simulink model "final simulation file"  (R2021a)
settings: Solver=ode8  StartTime=0.0  StopTime=0.1  FixedStep=1e-7  RelTol=1e-3
undefined symbols (not defined in the file): Acid, Lead
libraries: spsSeriesRLCBranchLib x13, spsIGBTLib x6, pid_lib x4, sldrtlib x4, spsAlphaBetaZerotodq0Lib x2, simulink x2, spsThreePhaseVIMeasurementLib x2, spsDiodeLib x1, spsIdealSwitchLib x1, spsMosfetLib x1, spsPower3phInstantaneousLib x1, spsBatteryLib x1
settings Model: Creator=RISHABH KUMAR  LastModifiedBy=RISHABH KUMAR

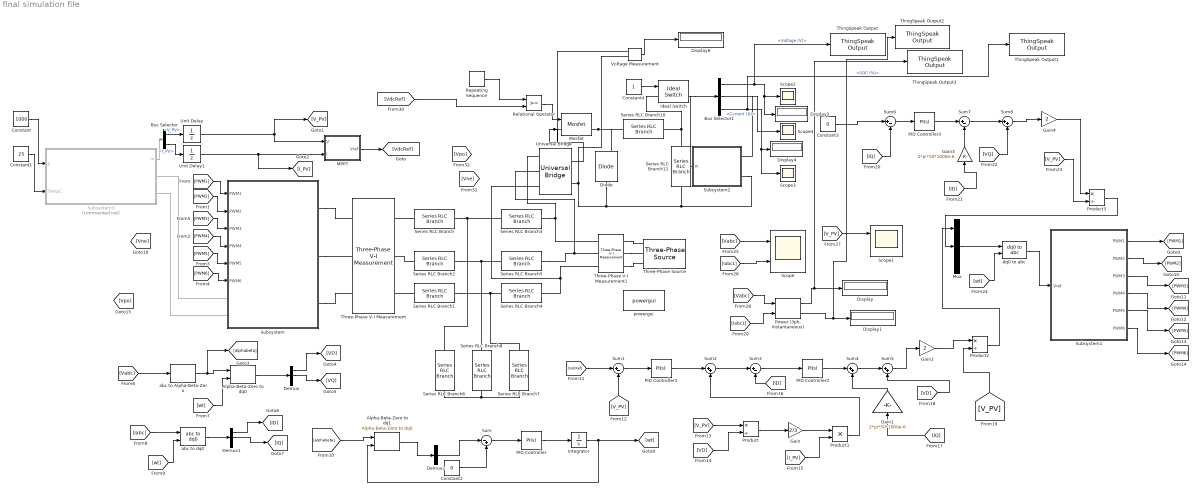
== system final simulation file ==
  Alpha-Beta-Zero to dq0 : spsAlphaBetaZerotodq0Lib/Alpha-Beta-Zero to dq0  Alignment=90 degrees behind phase A axis
      settings: SourceProductBaseCode=PS
  Alpha-Beta-Zero to dq1 : spsAlphaBetaZerotodq0Lib/Alpha-Beta-Zero to dq0  Alignment=90 degrees behind phase A axis
      settings: SourceProductBaseCode=PS
  Bus Selector : BusSelector  OutputSignals=V_PV,I_PV
  Bus Selector1 : BusSelector  OutputSignals=Voltage (V),Current (A),SOC (%)
  Constant : Constant  Value=1000
  Constant1 : Constant  Value=25
  Constant2 : Constant  Value=0
  Constant3 : Constant  Value=0
  Constant4 : Constant
  Demux : Demux  Outputs=3
  Demux1 : Demux  Outputs=3
  Demux2 : Demux  Outputs=3
  Diode : spsDiodeLib/Diode  Ron=0.001  Lon=0  Vf=0.8  IC=0  UseSnubber=0  Rs=500  Cs=250e-9  Measurements=on
  Display{,1..2,4,6} (5 alike) : Display
  Gain : Gain  Gain=2/3
  Gain1 : Gain  Gain=2*pi*50*1000e-6
  Gain2 : Gain  Gain=2
  Gain3 : Gain  Gain=2*pi*50*1000e-6
  Gain4 : Gain  Gain=2
  Ideal Switch : spsIdealSwitchLib/Ideal Switch  Ron=0.00001  Lon=0  IC=0  Rs=1e5  Cs=inf  Measurements=on
  Integrator : Integrator
  MPPT : MATLAB Function  TreatAsAtomicUnit=on
  Mosfet : spsMosfetLib/Mosfet  Ron=0.1  Lon=0  Rd=0.01  Vfd=0  IC=0  Rs=1e5  Cs=inf  Measurements=on
  Mux : Mux  Inputs=3
  PID Controller : pid_lib/PID Controller  Controller=PI  Form=Parallel  TimeDomain=Continuous-time  UseExternalTs=off  SampleTime=-1  IntegratorMethod=Forward Euler  FilterMethod=Forward Euler  ControllerParametersSource=internal  P=10  I=50000  D=0  UseFilter=on  N=100  TunerSelectOption=Transfer Function Based (PID Tuner App)  InitialConditionSource=internal  InitialConditionForIntegrator=0  InitialConditionForFilter=0  DifferentiatorICPrevScaledInput=0  ExternalReset=none  TrackingMode=off  Kt=1  LimitOutput=off  SatLimitsSource=internal  UpperSaturationLimit=inf  LowerSaturationLimit=-inf  LinearizeAsGain=on  AntiWindupMode=none  Kb=1  POutMin=[]  POutMax=[]  IOutMin=[]  IOutMax=[]  DOutMin=[]  DOutMax=[]  NOutMin=[]  NOutMax=[]  SumOutMin=[]  SumOutMax=[]  SaturationOutMin=[]  SaturationOutMax=[]  PParamMin=[]  PParamMax=[]  IParamMin=[]  IParamMax=[]  DParamMin=[]  DParamMax=[]  NParamMin=[]  NParamMax=[]  KbParamMin=[]  KbParamMax=[]  KtParamMin=[]  KtParamMax=[]  KbOutMin=[]  KbOutMax=[]  KtOutMin=[]  KtOutMax=[]  IntegratorOutMin=[]  IntegratorOutMax=[]  FilterOutMin=[]  FilterOutMax=[]  SumI1OutMin=[]  SumI1OutMax=[]  SumI2OutMin=[]  SumI2OutMax=[]  SumI3OutMin=[]  SumI3OutMax=[]  SumI4OutMin=[]  SumI4OutMax=[]  SumDOutMin=[]  SumDOutMax=[]  DifferentiatorOutMin=[]  DifferentiatorOutMax=[]  FilterDiffOutCoefMin=[]  FilterDiffOutCoefMax=[]  ReciprocalOutMin=[]  ReciprocalOutMax=[]  SumDenOutMin=[]  SumDenOutMax=[]  SumNumOutMin=[]  SumNumOutMax=[]  DivideOutMin=[]  DivideOutMax=[]  UdiffTsProdOutMin=[]  UdiffTsProdOutMax=[]  NTsProdOutMin=[]  NTsProdOutMax=[]  UintegralTsProdOutMin=[]  UintegralTsProdOutMax=[]  UngainTsProdOutMin=[]  UngainTsProdOutMax=[]  IntegratorContinuousStateAttributes=''  IntegratorStateMustResolveToSignalObject=off  IntegratorRTWStateStorageClass=Auto  FilterContinuousStateAttributes=''  FilterStateMustResolveToSignalObject=off  FilterRTWStateStorageClass=Auto  ParallelPVariant=InternalParameters  IdealPVariant=Disabled  IVariant=InternalParameters  DVariant=Disabled  IntegratorVariant=Continuous  SatVariant=Disabled  AWVariant=Passthrough  PCopyVariant=Disabled  TRVariant=Disabled  FdbkBlocksVariant=Forward  IdealPFdbkVariant=Disabled  SatFdbkVariant=Disabled  DerivativeFilterVariant=Disabled  NVariant=Disabled  NCopyVariant=Disabled_SignalSpec  FilterICVariant=Disabled  IntegratorICVariant=InternalICs  ExternalResetVariant=Disabled  TRSumVariant=Passthrough  SumFdbkVariant=Disabled  SumVariant=Sum_PI  TsampFilterVariant=InternalTs  TsampNgainVariant=Passthrough  TsampIntegralVariant=Passthrough  ExternalSaturationOutDataTypeStr=Inherit: Same as second input
  PID Controller1 : pid_lib/PID Controller  Controller=PI  Form=Parallel  TimeDomain=Continuous-time  UseExternalTs=off  SampleTime=-1  IntegratorMethod=Forward Euler  FilterMethod=Forward Euler  ControllerParametersSource=internal  P=0.25  I=0.001  D=0  UseFilter=on  N=100  TunerSelectOption=Transfer Function Based (PID Tuner App)  InitialConditionSource=internal  InitialConditionForIntegrator=0  InitialConditionForFilter=0  DifferentiatorICPrevScaledInput=0  ExternalReset=none  TrackingMode=off  Kt=1  LimitOutput=off  SatLimitsSource=internal  UpperSaturationLimit=inf  LowerSaturationLimit=-inf  LinearizeAsGain=on  AntiWindupMode=none  Kb=1  POutMin=[]  POutMax=[]  IOutMin=[]  IOutMax=[]  DOutMin=[]  DOutMax=[]  NOutMin=[]  NOutMax=[]  SumOutMin=[]  SumOutMax=[]  SaturationOutMin=[]  SaturationOutMax=[]  PParamMin=[]  PParamMax=[]  IParamMin=[]  IParamMax=[]  DParamMin=[]  DParamMax=[]  NParamMin=[]  NParamMax=[]  KbParamMin=[]  KbParamMax=[]  KtParamMin=[]  KtParamMax=[]  KbOutMin=[]  KbOutMax=[]  KtOutMin=[]  KtOutMax=[]  IntegratorOutMin=[]  IntegratorOutMax=[]  FilterOutMin=[]  FilterOutMax=[]  SumI1OutMin=[]  SumI1OutMax=[]  SumI2OutMin=[]  SumI2OutMax=[]  SumI3OutMin=[]  SumI3OutMax=[]  SumI4OutMin=[]  SumI4OutMax=[]  SumDOutMin=[]  SumDOutMax=[]  DifferentiatorOutMin=[]  DifferentiatorOutMax=[]  FilterDiffOutCoefMin=[]  FilterDiffOutCoefMax=[]  ReciprocalOutMin=[]  ReciprocalOutMax=[]  SumDenOutMin=[]  SumDenOutMax=[]  SumNumOutMin=[]  SumNumOutMax=[]  DivideOutMin=[]  DivideOutMax=[]  UdiffTsProdOutMin=[]  UdiffTsProdOutMax=[]  NTsProdOutMin=[]  NTsProdOutMax=[]  UintegralTsProdOutMin=[]  UintegralTsProdOutMax=[]  UngainTsProdOutMin=[]  UngainTsProdOutMax=[]  IntegratorContinuousStateAttributes=''  IntegratorStateMustResolveToSignalObject=off  IntegratorRTWStateStorageClass=Auto  FilterContinuousStateAttributes=''  FilterStateMustResolveToSignalObject=off  FilterRTWStateStorageClass=Auto  ParallelPVariant=InternalParameters  IdealPVariant=Disabled  IVariant=InternalParameters  DVariant=Disabled  IntegratorVariant=Continuous  SatVariant=Disabled  AWVariant=Passthrough  PCopyVariant=Disabled  TRVariant=Disabled  FdbkBlocksVariant=Forward  IdealPFdbkVariant=Disabled  SatFdbkVariant=Disabled  DerivativeFilterVariant=Disabled  NVariant=Disabled  NCopyVariant=Disabled_SignalSpec  FilterICVariant=Disabled  IntegratorICVariant=InternalICs  ExternalResetVariant=Disabled  TRSumVariant=Passthrough  SumFdbkVariant=Disabled  SumVariant=Sum_PI  TsampFilterVariant=InternalTs  TsampNgainVariant=Passthrough  TsampIntegralVariant=Passthrough  ExternalSaturationOutDataTypeStr=Inherit: Same as second input
  PID Controller2 : pid_lib/PID Controller  Controller=PI  Form=Parallel  TimeDomain=Continuous-time  UseExternalTs=off  SampleTime=-1  IntegratorMethod=Forward Euler  FilterMethod=Forward Euler  ControllerParametersSource=internal  P=3.33  I=5000  D=0  UseFilter=on  N=100  TunerSelectOption=Transfer Function Based (PID Tuner App)  InitialConditionSource=internal  InitialConditionForIntegrator=0  InitialConditionForFilter=0  DifferentiatorICPrevScaledInput=0  ExternalReset=none  TrackingMode=off  Kt=1  LimitOutput=off  SatLimitsSource=internal  UpperSaturationLimit=inf  LowerSaturationLimit=-inf  LinearizeAsGain=on  AntiWindupMode=none  Kb=1  POutMin=[]  POutMax=[]  IOutMin=[]  IOutMax=[]  DOutMin=[]  DOutMax=[]  NOutMin=[]  NOutMax=[]  SumOutMin=[]  SumOutMax=[]  SaturationOutMin=[]  SaturationOutMax=[]  PParamMin=[]  PParamMax=[]  IParamMin=[]  IParamMax=[]  DParamMin=[]  DParamMax=[]  NParamMin=[]  NParamMax=[]  KbParamMin=[]  KbParamMax=[]  KtParamMin=[]  KtParamMax=[]  KbOutMin=[]  KbOutMax=[]  KtOutMin=[]  KtOutMax=[]  IntegratorOutMin=[]  IntegratorOutMax=[]  FilterOutMin=[]  FilterOutMax=[]  SumI1OutMin=[]  SumI1OutMax=[]  SumI2OutMin=[]  SumI2OutMax=[]  SumI3OutMin=[]  SumI3OutMax=[]  SumI4OutMin=[]  SumI4OutMax=[]  SumDOutMin=[]  SumDOutMax=[]  DifferentiatorOutMin=[]  DifferentiatorOutMax=[]  FilterDiffOutCoefMin=[]  FilterDiffOutCoefMax=[]  ReciprocalOutMin=[]  ReciprocalOutMax=[]  SumDenOutMin=[]  SumDenOutMax=[]  SumNumOutMin=[]  SumNumOutMax=[]  DivideOutMin=[]  DivideOutMax=[]  UdiffTsProdOutMin=[]  UdiffTsProdOutMax=[]  NTsProdOutMin=[]  NTsProdOutMax=[]  UintegralTsProdOutMin=[]  UintegralTsProdOutMax=[]  UngainTsProdOutMin=[]  UngainTsProdOutMax=[]  IntegratorContinuousStateAttributes=''  IntegratorStateMustResolveToSignalObject=off  IntegratorRTWStateStorageClass=Auto  FilterContinuousStateAttributes=''  FilterStateMustResolveToSignalObject=off  FilterRTWStateStorageClass=Auto  ParallelPVariant=InternalParameters  IdealPVariant=Disabled  IVariant=InternalParameters  DVariant=Disabled  IntegratorVariant=Continuous  SatVariant=Disabled  AWVariant=Passthrough  PCopyVariant=Disabled  TRVariant=Disabled  FdbkBlocksVariant=Forward  IdealPFdbkVariant=Disabled  SatFdbkVariant=Disabled  DerivativeFilterVariant=Disabled  NVariant=Disabled  NCopyVariant=Disabled_SignalSpec  FilterICVariant=Disabled  IntegratorICVariant=InternalICs  ExternalResetVariant=Disabled  TRSumVariant=Passthrough  SumFdbkVariant=Disabled  SumVariant=Sum_PI  TsampFilterVariant=InternalTs  TsampNgainVariant=Passthrough  TsampIntegralVariant=Passthrough  ExternalSaturationOutDataTypeStr=Inherit: Same as second input
  PID Controller3 : pid_lib/PID Controller  Controller=PI  Form=Parallel  TimeDomain=Continuous-time  UseExternalTs=off  SampleTime=-1  IntegratorMethod=Forward Euler  FilterMethod=Forward Euler  ControllerParametersSource=internal  P=3.33  I=5000  D=0  UseFilter=on  N=100  TunerSelectOption=Transfer Function Based (PID Tuner App)  InitialConditionSource=internal  InitialConditionForIntegrator=0  InitialConditionForFilter=0  DifferentiatorICPrevScaledInput=0  ExternalReset=none  TrackingMode=off  Kt=1  LimitOutput=off  SatLimitsSource=internal  UpperSaturationLimit=inf  LowerSaturationLimit=-inf  LinearizeAsGain=on  AntiWindupMode=none  Kb=1  POutMin=[]  POutMax=[]  IOutMin=[]  IOutMax=[]  DOutMin=[]  DOutMax=[]  NOutMin=[]  NOutMax=[]  SumOutMin=[]  SumOutMax=[]  SaturationOutMin=[]  SaturationOutMax=[]  PParamMin=[]  PParamMax=[]  IParamMin=[]  IParamMax=[]  DParamMin=[]  DParamMax=[]  NParamMin=[]  NParamMax=[]  KbParamMin=[]  KbParamMax=[]  KtParamMin=[]  KtParamMax=[]  KbOutMin=[]  KbOutMax=[]  KtOutMin=[]  KtOutMax=[]  IntegratorOutMin=[]  IntegratorOutMax=[]  FilterOutMin=[]  FilterOutMax=[]  SumI1OutMin=[]  SumI1OutMax=[]  SumI2OutMin=[]  SumI2OutMax=[]  SumI3OutMin=[]  SumI3OutMax=[]  SumI4OutMin=[]  SumI4OutMax=[]  SumDOutMin=[]  SumDOutMax=[]  DifferentiatorOutMin=[]  DifferentiatorOutMax=[]  FilterDiffOutCoefMin=[]  FilterDiffOutCoefMax=[]  ReciprocalOutMin=[]  ReciprocalOutMax=[]  SumDenOutMin=[]  SumDenOutMax=[]  SumNumOutMin=[]  SumNumOutMax=[]  DivideOutMin=[]  DivideOutMax=[]  UdiffTsProdOutMin=[]  UdiffTsProdOutMax=[]  NTsProdOutMin=[]  NTsProdOutMax=[]  UintegralTsProdOutMin=[]  UintegralTsProdOutMax=[]  UngainTsProdOutMin=[]  UngainTsProdOutMax=[]  IntegratorContinuousStateAttributes=''  IntegratorStateMustResolveToSignalObject=off  IntegratorRTWStateStorageClass=Auto  FilterContinuousStateAttributes=''  FilterStateMustResolveToSignalObject=off  FilterRTWStateStorageClass=Auto  ParallelPVariant=InternalParameters  IdealPVariant=Disabled  IVariant=InternalParameters  DVariant=Disabled  IntegratorVariant=Continuous  SatVariant=Disabled  AWVariant=Passthrough  PCopyVariant=Disabled  TRVariant=Disabled  FdbkBlocksVariant=Forward  IdealPFdbkVariant=Disabled  SatFdbkVariant=Disabled  DerivativeFilterVariant=Disabled  NVariant=Disabled  NCopyVariant=Disabled_SignalSpec  FilterICVariant=Disabled  IntegratorICVariant=InternalICs  ExternalResetVariant=Disabled  TRSumVariant=Passthrough  SumFdbkVariant=Disabled  SumVariant=Sum_PI  TsampFilterVariant=InternalTs  TsampNgainVariant=Passthrough  TsampIntegralVariant=Passthrough  ExternalSaturationOutDataTypeStr=Inherit: Same as second input
  "Power (3ph, Instantaneous)" : spsPower3phInstantaneousLib/Power (3ph, Instantaneous)
  Product : Product  Inputs=*/
  Product1 : Product
  Product2 : Product  Inputs=*/
  Product3 : Product  Inputs=*/
  Relational Operator : RelationalOperator  OutDataTypeStr=boolean  RndMeth=Simplest
  Repeating Sequence : simulink/Sources/Repeating Sequence  rep_seq_t=[0 0.0001]  rep_seq_y=[0 1]
  Scope : Scope  NumInputPorts=2
  Scope1 : Scope  NumInputPorts=2
  Scope2 : Scope
  Scope3 : Scope
  Scope4 : Scope
  Series RLC Branch{,1..5} (6 alike) : spsSeriesRLCBranchLib/Series RLC Branch  LConnTagsString=__new0  RConnTagsString=__new0  BranchType=RL  Resistance=1e-3  Inductance=500e-3  SetiL0=off  InitialCurrent=0  Capacitance=1e-6  Setx0=off  InitialVoltage=0  Measurements=None
  Series RLC Branch10 : spsSeriesRLCBranchLib/Series RLC Branch  LConnTagsString=__new0  RConnTagsString=__new0  BranchType=L  Resistance=1  Inductance=0.0417  SetiL0=off  InitialCurrent=0  Capacitance=1e-6  Setx0=off  InitialVoltage=0  Measurements=None
  Series RLC Branch11 : spsSeriesRLCBranchLib/Series RLC Branch  LConnTagsString=__new0  RConnTagsString=__new0  BranchType=C  Resistance=1  Inductance=0.783e-3  SetiL0=off  InitialCurrent=0  Capacitance=1.198e-3  Setx0=off  InitialVoltage=0  Measurements=None
  Series RLC Branch6 : spsSeriesRLCBranchLib/Series RLC Branch  LConnTagsString=__new0  RConnTagsString=__new0  BranchType=RC  Resistance=1e-3  Inductance=500e-3  SetiL0=off  InitialCurrent=0  Capacitance=100e-6  Setx0=off  InitialVoltage=0  Measurements=None
  Series RLC Branch7 : spsSeriesRLCBranchLib/Series RLC Branch  LConnTagsString=__new0  RConnTagsString=__new0  BranchType=RC  Resistance=1e-3  Inductance=500e-3  SetiL0=off  InitialCurrent=0  Capacitance=100e-6  Setx0=off  InitialVoltage=0  Measurements=None
  Series RLC Branch8 : spsSeriesRLCBranchLib/Series RLC Branch  LConnTagsString=__new0  RConnTagsString=__new0  BranchType=RC  Resistance=1e-3  Inductance=500e-3  SetiL0=off  InitialCurrent=0  Capacitance=100e-6  Setx0=off  InitialVoltage=0  Measurements=None
  Subsystem : Subsystem
  Subsystem1 : Subsystem
  Subsystem2 : Subsystem
      mask Display: image('Red.jpg'); % Use "Edit Image" on toolstrip to change.
  Subsystem3 : Subsystem  Commented=on
      mask Display: image('C:\Users\RISHABH KUMAR\Downloads\adani solar panel logo - Google Search_files\Adani-Solar footer.png'); % Use "Edit Image" on toolstrip to change.
  Sum : Sum  Inputs=|-+
  Sum{1,3,6..7} (4 alike) : Sum  Inputs=|+-
  Sum{2,4..5,8} (4 alike) : Sum  Inputs=|++
  ThingSpeak Output : sldrtlib/Internet of Things/ThingSpeak Output  DrvAddress=1487592  DrvOptions=[1 20 50 49 54 54 82 88 71 90 70 83 87 72 74 54 56 66 97 112 105 46 116 104 105 110 103 115 112 101 97 107 46 99 111 109 0 0 0 0 0 0 0 0 0 0 0 0 0 0 0 0 0 0 0 0 0 0 0 0 0 0 0 0 0 0 0 0 0 0 0 0 0 0 0 0 0 0 0 0 0 0 0 0 0 0 0 0 0 0 0 0 0 0 0 0 0 0 0 0 0 0 0 0 0 0 0 0 0 0 0 0 0 0 0 0 0 0 0 0 0 0 0 0 0 0 0 0 0 0 0 0 0 0 0 0 0 0 0 0 0 0 0 0 0 0 0 0 0 0 0 0 0 0 0 0 0 0 0 0 0 0 0 0 0 0 0 0 0 0 0 0 0 0 0 0 0 0 0 0 0 0 0 0 0 0 0 0 0 0 0 0 0 0 0 0 0 0 0 0 0 0 0 0 0 0 0 0 0 0 0 0 0 0 0 0 0 0 0 0 0 0 0 0 0 0 0 0 0 0 0 0 0 0 0 0 0 0 0 0 0 0 0 0 0 0 0 0 0 0 0 0 0 0 0 0]  SampleTime=0.001  MaxMissedTicks=1000000000  ShowMissedTicks=off  YieldWhenWaiting=off  ChannelFields=1  OptParam=0  InitialValue=[]  FinalValue=[]
      settings: SourceProductBaseCode=WT
  ThingSpeak Output1 : sldrtlib/Internet of Things/ThingSpeak Output  DrvAddress=1487592  DrvOptions=[1 20 50 49 54 54 82 88 71 90 70 83 87 72 74 54 56 66 97 112 105 46 116 104 105 110 103 115 112 101 97 107 46 99 111 109 0 0 0 0 0 0 0 0 0 0 0 0 0 0 0 0 0 0 0 0 0 0 0 0 0 0 0 0 0 0 0 0 0 0 0 0 0 0 0 0 0 0 0 0 0 0 0 0 0 0 0 0 0 0 0 0 0 0 0 0 0 0 0 0 0 0 0 0 0 0 0 0 0 0 0 0 0 0 0 0 0 0 0 0 0 0 0 0 0 0 0 0 0 0 0 0 0 0 0 0 0 0 0 0 0 0 0 0 0 0 0 0 0 0 0 0 0 0 0 0 0 0 0 0 0 0 0 0 0 0 0 0 0 0 0 0 0 0 0 0 0 0 0 0 0 0 0 0 0 0 0 0 0 0 0 0 0 0 0 0 0 0 0 0 0 0 0 0 0 0 0 0 0 0 0 0 0 0 0 0 0 0 0 0 0 0 0 0 0 0 0 0 0 0 0 0 0 0 0 0 0 0 0 0 0 0 0 0 0 0 0 0 0 0 0 0 0 0 0 0]  SampleTime=0.001  MaxMissedTicks=1000000000  ShowMissedTicks=off  YieldWhenWaiting=off  ChannelFields=3  OptParam=0  InitialValue=[]  FinalValue=[]
      settings: SourceProductBaseCode=WT
  ThingSpeak Output2 : sldrtlib/Internet of Things/ThingSpeak Output  DrvAddress=1487592  DrvOptions=[1 20 50 49 54 54 82 88 71 90 70 83 87 72 74 54 56 66 97 112 105 46 116 104 105 110 103 115 112 101 97 107 46 99 111 109 0 0 0 0 0 0 0 0 0 0 0 0 0 0 0 0 0 0 0 0 0 0 0 0 0 0 0 0 0 0 0 0 0 0 0 0 0 0 0 0 0 0 0 0 0 0 0 0 0 0 0 0 0 0 0 0 0 0 0 0 0 0 0 0 0 0 0 0 0 0 0 0 0 0 0 0 0 0 0 0 0 0 0 0 0 0 0 0 0 0 0 0 0 0 0 0 0 0 0 0 0 0 0 0 0 0 0 0 0 0 0 0 0 0 0 0 0 0 0 0 0 0 0 0 0 0 0 0 0 0 0 0 0 0 0 0 0 0 0 0 0 0 0 0 0 0 0 0 0 0 0 0 0 0 0 0 0 0 0 0 0 0 0 0 0 0 0 0 0 0 0 0 0 0 0 0 0 0 0 0 0 0 0 0 0 0 0 0 0 0 0 0 0 0 0 0 0 0 0 0 0 0 0 0 0 0 0 0 0 0 0 0 0 0 0 0 0 0 0 0]  SampleTime=0.001  MaxMissedTicks=1000000000  ShowMissedTicks=off  YieldWhenWaiting=off  ChannelFields=2  OptParam=0  InitialValue=[]  FinalValue=[]
      settings: SourceProductBaseCode=WT
  ThingSpeak Output3 : sldrtlib/Internet of Things/ThingSpeak Output  DrvAddress=1487592  DrvOptions=[1 20 50 49 54 54 82 88 71 90 70 83 87 72 74 54 56 66 97 112 105 46 116 104 105 110 103 115 112 101 97 107 46 99 111 109 0 0 0 0 0 0 0 0 0 0 0 0 0 0 0 0 0 0 0 0 0 0 0 0 0 0 0 0 0 0 0 0 0 0 0 0 0 0 0 0 0 0 0 0 0 0 0 0 0 0 0 0 0 0 0 0 0 0 0 0 0 0 0 0 0 0 0 0 0 0 0 0 0 0 0 0 0 0 0 0 0 0 0 0 0 0 0 0 0 0 0 0 0 0 0 0 0 0 0 0 0 0 0 0 0 0 0 0 0 0 0 0 0 0 0 0 0 0 0 0 0 0 0 0 0 0 0 0 0 0 0 0 0 0 0 0 0 0 0 0 0 0 0 0 0 0 0 0 0 0 0 0 0 0 0 0 0 0 0 0 0 0 0 0 0 0 0 0 0 0 0 0 0 0 0 0 0 0 0 0 0 0 0 0 0 0 0 0 0 0 0 0 0 0 0 0 0 0 0 0 0 0 0 0 0 0 0 0 0 0 0 0 0 0 0 0 0 0 0 0]  SampleTime=0.001  MaxMissedTicks=1000000000  ShowMissedTicks=off  YieldWhenWaiting=off  ChannelFields=4  OptParam=0  InitialValue=[]  FinalValue=[]
      settings: SourceProductBaseCode=WT
  Three-Phase V-I Measurement : spsThreePhaseVIMeasurementLib/Three-Phase V-I Measurement  VoltageMeasurement=no  SetLabelV=off  LabelV=Vabc  Vpu=off  VpuLL=off  CurrentMeasurement=yes  SetLabelI=on  LabelI=Iabc  Ipu=off  Pbase=100e6  Vbase=500e3  OutputType=Complex  PhasorSimulation=off  PSBequivalent=0
  Three-Phase V-I Measurement1 : spsThreePhaseVIMeasurementLib/Three-Phase V-I Measurement  VoltageMeasurement=phase-to-ground  SetLabelV=on  LabelV=Vabc  Vpu=off  VpuLL=off  CurrentMeasurement=yes  SetLabelI=on  LabelI=Iabc1  Ipu=off  Pbase=100e6  Vbase=500e3  OutputType=Complex  PhasorSimulation=off  PSBequivalent=0
  Three-Phase Source : spsThreePhaseSourceLib/Three-Phase Source  InternalConnection=Yg  VoltagePhases=off  Voltage=400  PhaseAngle=0  Voltage_phases=[25e3 25e3 25e3]/sqrt(3)  PhaseAngles_phases=[0 -120 +120]  Frequency=50  NonIdealSource=on  SpecifyImpedance=off  Resistance=1e-6  Inductance=1e-6  ShortCircuitLevel=100e6  BaseVoltage=400  XRratio=7  BusType=swing  Pref=10e3  Qref=0  Prefabc=[10e3, 10e3, 10e3]  Qrefabc=[0, 0, 0]  Qmin=-inf  Qmax=inf
  Unit Delay : UnitDelay  SampleTime=1e-4  HasFrameUpgradeWarning=on
  Unit Delay1 : UnitDelay  SampleTime=1e-4  HasFrameUpgradeWarning=on
  Universal Bridge : spsUniversalBridgeLib/Universal Bridge  Arms=3  SnubberResistance=1e5  SnubberCapacitance=inf  Device=Diodes  Ron=1e-3  Lon=0  ForwardVoltages="[  0  0  ]"  ForwardVoltage=0  GTOparameters=[ 10e-6 , 20e-6 ]  IGBTparameters=[ 1e-6 , 2e-6 ]  Measurements=None  Measurements_2=None  converterType=Rectifier
  Voltage Measurement : spsVoltageMeasurementLib/Voltage Measurement  PhasorSimulation=off  OutputType=Complex  PSBequivalent=0
  abc to Alpha-Beta-Zero : spsabctoAlphaBetaZeroLib/abc to Alpha-Beta-Zero
      settings: SourceProductBaseCode=PS
  abc to dq0 : spsabctodq0Lib/abc to dq0  Alignment=90 degrees behind phase A axis
  dq0 to abc : spsdq0toabcLib/dq0 to abc  Alignment=90 degrees behind phase A axis
  powergui : spspowerguiLib/powergui  Priority=1  SimulationMode=Discrete  SampleTime=1e-7  frequency=60  Iterations=50  frequencyindice=0  Pbase=100e6  ErrMax=1e-4  UnitsV=kV  UnitsW=MW  buscounter=0  FunctionMessages=off  echomessages=off  EnableUseOfTLC=off  CurrentSourceSwitches=off  DisableSnubberDevices=off  DisableRonSwitches=off  DisableVfSwitches=off  DisplayEquations=off  AutomaticDiscreteSolvers=off  SolverType=Tustin/Backward Euler (TBE)  Interpol=off  ExternalGateDelay=off  methode=off  Ts=100  x0status=blocks  SPID=on  SwTol=0  HookPort=off  NonlinearTolerance=1e-4  nMaxIteration=100  ContinueOnMaxIteration=off  RestoreLinks=warning  ResistiveCurrentMeasurement=off  Frange=[0:2:500]  Ylog=off  Xlog=on  ShowGrid=off  save=off  variable=ZData  structure=0  ZoomFFT=off  StartTime=0.0  cycles=1  DisplayStyle=1  fundamental=60  FreqAxis=off  MaxFrequency=1000  frequencyindicesteady=1  RmsSteady=1  display=off
  wires:
  Bus Selector/2 -> Unit Delay1/1  "<I_PV>"
  Bus Selector/1 -> Unit Delay/1  "<V_PV>"
  Unit Delay/1 -> [V_PV], MPPT/1(V)
  Unit Delay1/1 -> [I_PV], MPPT/2(I)
  MPPT/1(Vref) -> [VdcRef]
  [PWM1] -> Subsystem/1(PWM1)
  [PWM6] -> Subsystem/6(PWM6)
  [PWM5] -> Subsystem/5(PWM5)
  [PWM4] -> Subsystem/4(PWM4)
  [PWM3] -> Subsystem/3(PWM3)
  [PWM2] -> Subsystem/2(PWM2)
  [Vabc] -> abc to Alpha-Beta-Zero/1
  abc to Alpha-Beta-Zero/1 -> [alphabeta], Alpha-Beta-Zero to dq0/1
  [wt] -> Alpha-Beta-Zero to dq0/2
  Alpha-Beta-Zero to dq0/1 -> Demux/1
  Demux/1 -> [VD]
  Demux/2 -> [VQ]
  [Iabc] -> abc to dq0/1
  [wt] -> abc to dq0/2
  abc to dq0/1 -> Demux1/1
  Demux1/1 -> [ID]
  Demux1/2 -> [IQ]
  [alphabeta] -> Alpha-Beta-Zero to dq1/1
  Alpha-Beta-Zero to dq1/1 -> Demux2/1
  Demux2/2 -> Sum/1
  Constant2/1 -> Sum/2
  Sum/1 -> PID Controller/1
  PID Controller/1 -> Integrator/1
  Integrator/1 -> [wt], Alpha-Beta-Zero to dq1/2
  [VdcRef] -> Sum1/1
  [V_PV] -> Sum1/2
  Sum1/1 -> PID Controller1/1
  PID Controller1/1 -> Sum2/1
  [V_PV] -> Product/1
  [VD] -> Product/2
  Product/1 -> Gain/1
  Gain/1 -> Product1/1
  [I_PV] -> Product1/2
  Product1/1 -> Sum2/2
  Sum2/1 -> Sum3/1
  [ID] -> Sum3/2
  Sum3/1 -> PID Controller2/1
  PID Controller2/1 -> Sum4/1
  Gain1/1 -> Sum4/2
  [IQ] -> Gain1/1
  Sum4/1 -> Sum5/1
  [VD] -> Sum5/2
  Sum5/1 -> Gain2/1
  Gain2/1 -> Product2/1
  [V_PV] -> Product2/2
  Constant3/1 -> Sum6/1
  [IQ] -> Sum6/2
  Sum6/1 -> PID Controller3/1
  PID Controller3/1 -> Sum7/1
  Gain3/1 -> Sum7/2
  [ID] -> Gain3/1
  Sum7/1 -> Sum8/1
  [VQ] -> Sum8/2
  Sum8/1 -> Gain4/1
  Gain4/1 -> Product3/1
  [V_PV] -> Product3/2
  Product3/1 -> Mux/2
  Product2/1 -> Mux/1
  Mux/1 -> dq0 to abc/1
  [wt] -> dq0 to abc/2
  dq0 to abc/1 -> Subsystem1/1(Vref)
  Subsystem1/1(PWM1) -> [PWM1]
  Subsystem1/2(PWM2) -> [PWM2]
  Subsystem1/3(PWM3) -> [PWM3]
  Subsystem1/4(PWM4) -> [PWM4]
  Subsystem1/5(PWM5) -> [PWM5]
  Subsystem1/6(PWM6) -> [PWM6]
  [Vabc] -> Scope/1
  [Iabc1] -> Scope/2
  [V_PV] -> Scope1/1
  [Vabc] -> "Power (3ph, Instantaneous)"/1
  [Iabc1] -> "Power (3ph, Instantaneous)"/2
  "Power (3ph, Instantaneous)"/1 -> ThingSpeak Output3/1, Display/1
  "Power (3ph, Instantaneous)"/2 -> ThingSpeak Output2/1, Display1/1
  Voltage Measurement/1 -> Display6/1
  Bus Selector1/2 -> Scope4/1  "<Current (A)>"
  Relational Operator/1 -> Mosfet/1
  Bus Selector1/3 -> ThingSpeak Output1/1, Scope3/1, Display4/1  "<SOC (%)>"
  Bus Selector1/1 -> ThingSpeak Output/1, Scope2/1, Display2/1  "<Voltage (V)>"
  Repeating Sequence/1 -> Relational Operator/1
  [VdcRef] -> Relational Operator/2
  Constant4/1 -> Ideal Switch/1
  Subsystem2/1(m) -> Bus Selector1/1
  Constant/1 -> Subsystem3/1(S)
  Constant1/1 -> Subsystem3/2(TempC)
  Subsystem3/1(m) -> Bus Selector/1
  connections:
  Subsystem/RConn3 -- Three-Phase V-I Measurement/LConn3
  Subsystem/RConn2 -- Three-Phase V-I Measurement/LConn2
  Subsystem/RConn1 -- Three-Phase V-I Measurement/LConn1
  Series RLC Branch/LConn1 -- Three-Phase V-I Measurement/RConn1
  Series RLC Branch2/LConn1 -- Three-Phase V-I Measurement/RConn2
  Series RLC Branch1/LConn1 -- Three-Phase V-I Measurement/RConn3
  Series RLC Branch/RConn1 -- Series RLC Branch6/LConn1 -- Series RLC Branch3/LConn1
  Series RLC Branch2/RConn1 -- Series RLC Branch8/LConn1 -- Series RLC Branch5/LConn1
  Series RLC Branch1/RConn1 -- Series RLC Branch7/LConn1 -- Series RLC Branch4/LConn1
  Series RLC Branch6/RConn1 -- Series RLC Branch8/RConn1 -- Series RLC Branch7/RConn1
  Series RLC Branch3/RConn1 -- Universal Bridge/LConn1 -- Three-Phase V-I Measurement1/RConn1
  Series RLC Branch5/RConn1 -- Universal Bridge/LConn2 -- Three-Phase V-I Measurement1/RConn2
  Three-Phase V-I Measurement1/RConn3 -- Series RLC Branch4/RConn1 -- Universal Bridge/LConn3
  Three-Phase V-I Measurement1/LConn1 -- Three-Phase Source/RConn1
  Three-Phase V-I Measurement1/LConn2 -- Three-Phase Source/RConn2
  Three-Phase V-I Measurement1/LConn3 -- Three-Phase Source/RConn3
  Mosfet/LConn1 -- Universal Bridge/RConn1 -- Voltage Measurement/LConn1
  Universal Bridge/RConn2 -- Diode/LConn1 -- Subsystem2/LConn2 -- Series RLC Branch11/LConn1 -- Voltage Measurement/LConn2
  Mosfet/RConn1 -- Series RLC Branch10/RConn1 -- Diode/RConn1
  Series RLC Branch11/RConn1 -- Ideal Switch/LConn1 -- Series RLC Branch10/LConn1
  Ideal Switch/RConn1 -- Subsystem2/LConn1
  Subsystem3/RConn1 -- Subsystem/LConn1
  Subsystem3/RConn2 -- Subsystem/LConn2

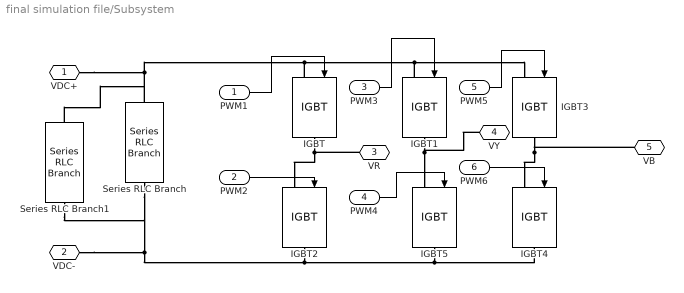
== system final simulation file/Subsystem ==
  PWM1 : Inport
  PWM2 : Inport  Port=2
  PWM3 : Inport  Port=3
  PWM4 : Inport  Port=4
  PWM5 : Inport  Port=5
  PWM6 : Inport  Port=6
  IGBT{,1..5} (6 alike) : spsIGBTLib/IGBT  Ron=0.001  Lon=0  Vf=1  Tf=1e-6  Tt=2e-6  IC=0  Rs=1e5  Cs=inf  Measurements=off
  Series RLC Branch : spsSeriesRLCBranchLib/Series RLC Branch  LConnTagsString=__new0  RConnTagsString=__new0  BranchType=RC  Resistance=1e-3  Inductance=1e-3  SetiL0=off  InitialCurrent=0  Capacitance=500e-6  Setx0=off  InitialVoltage=0  Measurements=None
  Series RLC Branch1 : spsSeriesRLCBranchLib/Series RLC Branch  LConnTagsString=__new0  RConnTagsString=__new0  BranchType=RC  Resistance=1e-3  Inductance=1e-3  SetiL0=off  InitialCurrent=0  Capacitance=500e-6  Setx0=off  InitialVoltage=0  Measurements=None
  VDC+ : PMIOPort  Side=Left
  VDC- : PMIOPort  Port=2  Side=Left
  VR : PMIOPort  Port=3  Side=Right
  VY : PMIOPort  Port=4  Side=Right
  VB : PMIOPort  Port=5  Side=Right
  wires:
  PWM3/1 -> IGBT1/1
  PWM1/1 -> IGBT/1
  PWM4/1 -> IGBT5/1
  PWM6/1 -> IGBT4/1
  PWM2/1 -> IGBT2/1
  PWM5/1 -> IGBT3/1
  connections:
  IGBT/RConn1 -- VR/RConn1 -- IGBT2/LConn1
  IGBT2/RConn1 -- Series RLC Branch1/RConn1 -- Series RLC Branch/RConn1 -- VDC-/RConn1 -- IGBT5/RConn1 -- IGBT4/RConn1
  IGBT1/RConn1 -- IGBT5/LConn1 -- VY/RConn1
  IGBT3/RConn1 -- VB/RConn1 -- IGBT4/LConn1
  IGBT/LConn1 -- Series RLC Branch1/LConn1 -- Series RLC Branch/LConn1 -- VDC+/RConn1 -- IGBT1/LConn1 -- IGBT3/LConn1

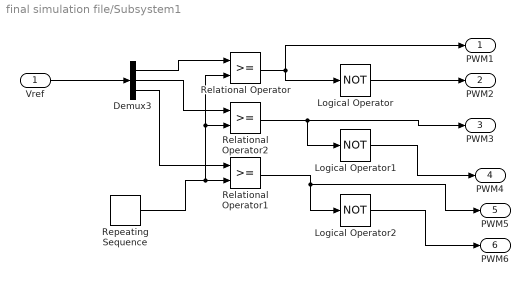
== system final simulation file/Subsystem1 ==
  Vref : Inport
  Demux3 : Demux  Outputs=3
  Logical Operator : Logic  Operator=NOT  AllPortsSameDT=off  OutDataTypeStr=boolean
  Logical Operator1 : Logic  Operator=NOT  AllPortsSameDT=off  OutDataTypeStr=boolean
  Logical Operator2 : Logic  Operator=NOT  AllPortsSameDT=off  OutDataTypeStr=boolean
  Relational Operator : RelationalOperator  OutDataTypeStr=boolean  RndMeth=Simplest
  Relational Operator1 : RelationalOperator  OutDataTypeStr=boolean  RndMeth=Simplest
  Relational Operator2 : RelationalOperator  OutDataTypeStr=boolean  RndMeth=Simplest
  Repeating Sequence : simulink/Sources/Repeating Sequence  rep_seq_t=[0 0.00005 0.0001]  rep_seq_y=[-1 1 -1]
  PWM1 : Outport
  PWM2 : Outport  Port=2
  PWM3 : Outport  Port=3
  PWM4 : Outport  Port=4
  PWM5 : Outport  Port=5
  PWM6 : Outport  Port=6
  wires:
  Demux3/1 -> Relational Operator/1
  Relational Operator/1 -> PWM1/1, Logical Operator/1
  Logical Operator2/1 -> PWM6/1
  Relational Operator1/1 -> PWM5/1, Logical Operator2/1
  Demux3/2 -> Relational Operator2/1
  Repeating Sequence/1 -> Relational Operator/2, Relational Operator2/2, Relational Operator1/2
  Vref/1 -> Demux3/1
  Relational Operator2/1 -> PWM3/1, Logical Operator1/1
  Demux3/3 -> Relational Operator1/1
  Logical Operator1/1 -> PWM4/1
  Logical Operator/1 -> PWM2/1

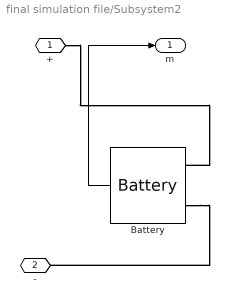
== system final simulation file/Subsystem2 ==
  Battery : spsBatteryLib/Battery  BatType=Lead-Acid  ShowTempParam=off  ThermalPreset=no  ShowAgeParam=off  NomV=100  NomQ=1000  SOC=45  Batt_Tr=1  PresetModel=on  MaxQ=1041.6667  MinV=75  FullV=108.8816  Dis_rate=200  R=0.001  Normal_OP=310.2778  expZone="[101.8092      3.333333]"  current=[6.5 13 32.5]  Units=Time  Tci=20  NomT=20  T2=-30  MaxQ2=4.8  FullV2=7.1  Normal_OP2=5.655  expZone2="[6.58           1]"  Rca=0.6  ti=2000  Dp=0  Neq0=0  Tsim=1e6  Ta1=25  Qeol=5.4*0.9  Reol=0.013333*1.2  Char_age=[2.3478, 3]  Dis_age=[2.3478, 10]  N1=1500  N2=10500  N3=1000  N4=1400  Ta2=45  N5=950
  + : PMIOPort  Side=Left
  - : PMIOPort  Port=2  Side=Left
  m : Outport
  wires:
  Battery/1 -> m/1
  connections:
  Battery/LConn2 -- -/RConn1
  +/RConn1 -- Battery/LConn1

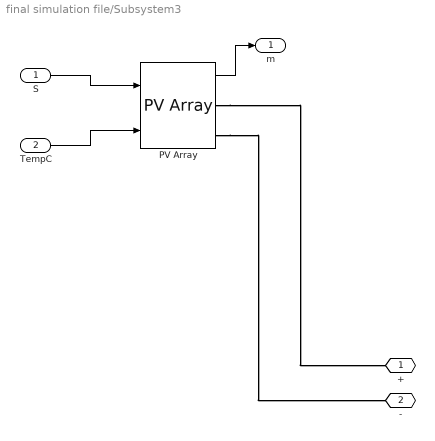
== system final simulation file/Subsystem3 ==
  S : Inport
  TempC : Inport  Port=2
  PV Array : spsPVArrayLib/PV Array  Npar=18  Nser=25  PlotType=array @ 25 deg.C & specified irradiances  S_vec="[ 1000  500  100 ]"  Temp_C_vec="[ 45 25  ]"  ModuleName=User-defined  PlotWhenSelected=off  Pm=213.15  Ncell=60  Voc=36.3  Isc=7.84  Vm=29  Im=7.35  beta_Voc_pc=-0.36099  alpha_Isc_pc=0.102  beta_Voc=-0.13104  alpha_Isc=0.0079968  IL=7.8654  I0=2.9273e-10  nI=0.98119  Rsh=313.0553  Rs=0.39381  RobustModel=off  RobustCellTemperature=313.3991  BAL=on  Tc=1e-6  Tfilter=5e-5
  + : PMIOPort  Side=Right
  - : PMIOPort  Port=2  Side=Right
  m : Outport
  wires:
  TempC/1 -> PV Array/2
  S/1 -> PV Array/1
  PV Array/1 -> m/1
  connections:
  PV Array/RConn1 -- +/RConn1
  PV Array/RConn2 -- -/RConn1

== matlab function final simulation file/MPPT ==
  data: V input; Vref output; I input
function Vref = RefGen(V,I)

Vrefmax = 907.5;
Vrefmin = 0;
Vrefinit = 750;
deltaVref = 1;
persistent Vold Pold Vrefold;

dataType = 'double';
if isempty(Vold)
    Vold = 0;
    Pold=0;
    Vrefold = Vrefinit;
end

P= V*I;
dV = V-Vold;
dP = P-Pold;

if dP ~= 0
    if dP<0
        if dV<0
            Vref = Vrefold + deltaVref;
        else
            Vref = Vrefold - deltaVref;
        end
    else
        if dV<0
            Vref = Vrefold - deltaVref;
        else
            Vref = Vrefold + deltaVref;
        end
    end
else
    Vref = Vrefold;
end
if Vref >= Vrefmax | Vref <= Vrefmin
    Vref = Vrefold;
end
Vrefold = Vref;
Vold = V;
Pold = P;
